simulink model "PlantaTFG2020a"  (R2020a)
settings: Solver=FixedStepAuto  StartTime=0.0  StopTime=30  FixedStep=0.001  RelTol=1e-3
values from neighbouring files (symbols this model uses):
  K = 61    [TFG_Preload.m]
  Kpot = 1.688    [TFG_Preload.m]
  Ktac = 0.01338    [TFG_Preload.m]
  tau = 0.293    [TFG_Preload.m]
  trueK = 61    [TFG_Preload.m]
undefined symbols (not defined in the file or in its folder): inputGain, inputOffset, inputType, Kd, Ki, Kp, loopType
libraries: simulink x1
settings Model: Creator=FactCore  LastModifiedBy=FactCore
settings DebuggingCC: SFMachineParentedDataDiag=error

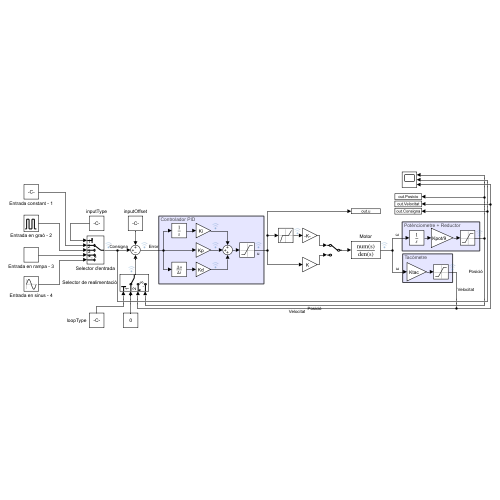
[thumbnail: Simulink's stored preview of the top-level diagram]
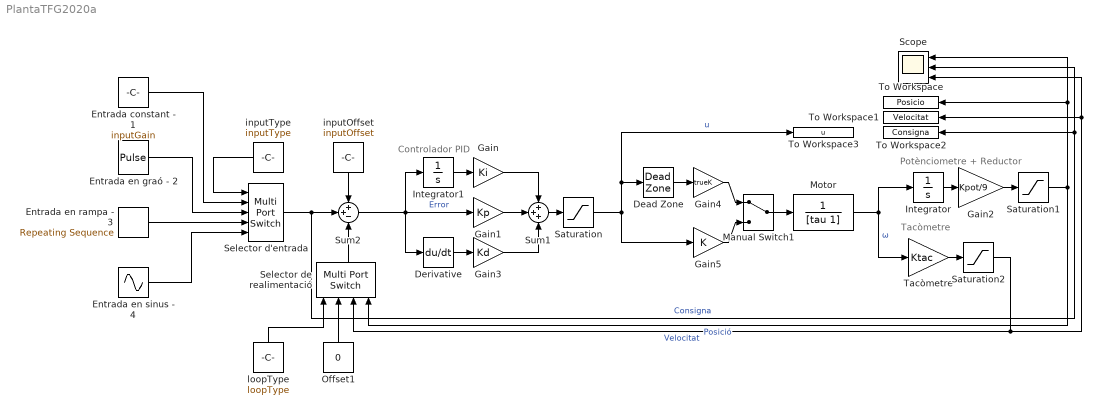
== system PlantaTFG2020a ==
  note: Controlador PID
  note: Tacòmetre
  note: Potènciometre + Reductor
  Dead Zone : DeadZone  LowerValue=Vdi  UpperValue=Vds  SaturateOnIntegerOverflow=on
  Derivative : Derivative
  Entrada constant - 1 : Constant  Value=inputGain
  Entrada en graó - 2 : DiscretePulseGenerator  PulseType=Time based  Amplitude=inputGain  Period=10  PulseWidth=50
  Entrada en rampa - 3 : simulink/Sources/Repeating Sequence  rep_seq_t=[0 10]  rep_seq_y=[0 inputGain]
  Entrada en sinus - 4 : Sin  Amplitude=inputGain*2  Frequency=2*pi*0.5  SampleTime=0
  Gain : Gain  Gain=Ki
  Gain1 : Gain  Gain=Kp
  Gain2 : Gain  Gain=Kpot/9
  Gain3 : Gain  Gain=Kd
  Gain4 : Gain  Gain=trueK
  Gain5 : Gain  Gain=K
  Integrator : Integrator
  Integrator1 : Integrator
  Manual Switch1 : ManualSwitch
  Motor : TransferFcn  Denominator=[tau 1]
  Offset1 : Constant  Value=0
  Saturation : Saturate  UpperLimit=5  LowerLimit=-5
  Saturation1 : Saturate  UpperLimit=5  LowerLimit=-5
  Saturation2 : Saturate  UpperLimit=5  LowerLimit=-5
  Scope : Scope  NumInputPorts=3
  Selector d'entrada : MultiPortSwitch  Inputs=4  OutDataTypeStr=single
  Selector de realimentació : MultiPortSwitch  OutDataTypeStr=single
  Sum1 : Sum  Inputs=+++
  Sum2 : Sum  Inputs=++-
  Tacòmetre : Gain  Gain=Ktac
  To Workspace : ToWorkspace  VariableName=Posicio  SaveFormat=Timeseries  SampleTime=-1
  To Workspace1 : ToWorkspace  VariableName=Velocitat  SaveFormat=Timeseries  SampleTime=-1
  To Workspace2 : ToWorkspace  VariableName=Consigna  SaveFormat=Timeseries  SampleTime=-1
  To Workspace3 : ToWorkspace  VariableName=u  SaveFormat=Timeseries  SampleTime=-1
  inputOffset : Constant  Value=inputOffset
  inputType : Constant  Value=inputType
  loopType : Constant  Value=loopType
  wires:
  Motor/1 -> Tacòmetre/1, Integrator/1  "ω"
  Sum2/1 -> Derivative/1, Integrator1/1, Gain1/1  "Error"
  Integrator/1 -> Gain2/1
  Integrator1/1 -> Gain/1
  Derivative/1 -> Gain3/1
  Gain/1 -> Sum1/1
  Gain3/1 -> Sum1/3
  Gain1/1 -> Sum1/2
  Sum1/1 -> Saturation/1
  inputType/1 -> Selector d'entrada/1
  Entrada en graó - 2/1 -> Selector d'entrada/3
  Entrada en rampa - 3/1 -> Selector d'entrada/4
  Entrada constant - 1/1 -> Selector d'entrada/2
  Selector d'entrada/1 -> Sum2/2, Scope/2, To Workspace2/1  "Consigna"
  Entrada en sinus - 4/1 -> Selector d'entrada/5
  inputOffset/1 -> Sum2/1
  Selector de realimentació/1 -> Sum2/3
  Gain2/1 -> Saturation1/1
  Manual Switch1/1 -> Motor/1
  Saturation/1 -> Gain5/1, To Workspace3/1, Dead Zone/1  "u"
  Gain5/1 -> Manual Switch1/2
  Dead Zone/1 -> Gain4/1
  Gain4/1 -> Manual Switch1/1
  Tacòmetre/1 -> Saturation2/1
  Saturation1/1 -> Selector de realimentació/4, Scope/1, To Workspace/1  "Posició"
  Saturation2/1 -> Selector de realimentació/3, To Workspace1/1, Scope/3  "Velocitat"
  Offset1/1 -> Selector de realimentació/2
  loopType/1 -> Selector de realimentació/1
